simulink model "Wanchao_Shuttlecock_New"  (Simulink 7.7)
settings: Solver=ode4  StartTime=0.0  StopTime=inf  FixedStep=sample_time  RelTol=1e-3
InitFcn:
  | sample_time=0.005;%0.004;%0.0025;%0.02;
  | DeltaT = 0.02;
  | g = 9.81;
  | H0 = g%0.3165;
  | Kl = 1;
  | 
  | Omega_r = 1.6;%for Horizontal reference
  | Zeta_r = 0.7; %for Horizontal reference
  | Omega = 1.8;%for Horizontal Control
  | Zeta = 0.5;    %for Horizontal Control
  | 
  | Omega_h_r = 2.5; %for vertical reference
  | Zeta_h_r = 0.8;  %for vertical reference
  | Omega_h = 2.7;    %for vertical control
  | Zeta_h = 0.8;         %for vertical control
  | PI=pi;
  | 
  | Mass = 1;
  | Acc_Max = 4;
  | Acc_Max_h = 4;
  | 
  | Max_RP = 60;
undefined symbols (not defined in the file or in its folder): DiscIntNeverNeededParam
libraries: simulink x7, dspadpt3 x3, X330_Control x2, X400_Control x1
(part 2 of 2)

== stateflow chart Planning/Trajectory Logic/UAV SF ==
  state Airborne
    state TakeOff
      du:HoverThrottle = (H0 - HoverThrottle)*3*DeltaT + HoverThrottle ;
    state Initialization
      du:PosDesired[0]=InitialPos[0];PosDesired[1]=InitialPos[1];
      PosDesired[2]=InitialPos[2];
    state SafyHover
      en:PosDesired = Pos; PosDesired[2]=-0.9;
    state Prelanding
      en:PosDesired[0]=InitialPos[0];PosDesired[1]=InitialPos[1];
      PosDesired[2]=InitialPos[2];
    state Descent
      en:PosDesired[2] = PerchPos[2]-0.15;
    state TrajE
      state OutputTargetPos
        en:PosDesired[0]=xp;
        PosDesired[1]=yp;
        PosDesired[2]=zp;
        dp[0]=xp;dp[1]=yp;dp[2]=zp;
      state DAQ
        en:i=0;DataReady=0;
        du:x[i]=Shuttlecock[0];[i]=Shuttlecock[1];
        z[i]=Shuttlecock[2];i++;
      state Estimation
        en:[xp,yp,zp,drz,rr]=TrajEst2(x,y,z,H);
      OutputTargetPos -> (junction 26)
      (default) -> DAQ
      Estimation -> OutputTargetPos [order 2] : [(abs(xp)<1)&(abs(yp+0.5)<1)]
      Estimation -> (junction 26) [order 1] : [(abs(xp)>=1)|(abs(yp+0.5)>=1)]
      DAQ -> Estimation : [i==5]
      (junction 26) -> DAQ [order 2] : [(Shuttlecock[2]-H<=-0.4)|(drz<0)]
    (default) -> TakeOff : {PosDesired = Pos;PosDesired[2] =-0.9;}
    TakeOff -> Initialization : after(1,sec)
    Initialization -> TrajE [order 1] : [(abs(Shuttlecock[0])<1)&(Shuttlecock[1]<2.5)&(Shuttlecock[2]<H-0.2)]
    Initialization -> SafyHover [order 2] : [RC[5] > 0]
    (junction 26) -> SafyHover [order 1] : [(RC[5] > 0)|((Shuttlecock[2]-H>-0.4)&(drz>=0))]
    SafyHover -> Prelanding : after(3, sec)
    Prelanding -> Descent : [PerchError < 0.01]
  state Landing
    state Descending
      en:PosDesired = Pos;
      du:PosDesired[2] = (PerchPos[2]- PosDesired[2])*1*DeltaT + PosDesired[2] ;
    state CutThrottle
      du:HoverThrottle = (0 - HoverThrottle)*3*DeltaT + HoverThrottle ;
    (default) -> Descending
    Descending -> CutThrottle : [Pos[2] > (PerchPos[2]-0.1)]
  (default) -> Airborne : {HoverThrottle = 0;}
  Landing -> Airborne : [RC[6] > 0.5]
  Airborne -> Landing : [RC[6] < -0.5]
  data: px function_input double size=5; py function_input double size=5; pz function_input double size=5; xe function_output double size=1; Hz function_input double size=1; ye function_output double size=1; ze function_output double size=1; zd function_output double size=1; p local double size=3 =[0 0 0]; t constant double size=5 =[0 0.02 0.04 0.06 0.08]; r function_output double; px function_input double size=5; py function_input double size=5; pz function_input double size=5; xe function_output double size=1; Hz function_input double size=1; ye function_output double size=1; ze function_output double size=1; zd function_output double size=1; x local double size=5 =[0 0 0 0 0]; y local double size=5 =[0 0 0 0 0]; z local double size=5 =[0 0 0 0 0]; xp local double; yp local double; zp local double; x_cache local double size=5 =[0 0 0 0 0]; y_cache local double size=5 =[0 0 0 0 0]; z_cache local double size=5 =[0 0 0 0 0]; px function_input double size=5; py function_input double size=5; pz function_input double size=5; xe function_output double size=1; Hz function_input double size=1; ye function_output double size=1; ze function_output double size=1; zd function_output double size=1; PosDesired output double size=4; HoverThrottle output double size=1; Mode output uint8 size=1; RC input double size=8; Pos input double size=4; PerchPos input double size=4; DeltaT parameter double size=1; H0 parameter double size=1; Kl parameter double size=1; VelCmd local double size=2 =0; PWM output double; PerchError input double; PI parameter double size=1; Shuttlecock input double size=3; H constant double =-1; InitialPos constant double size=3 =[0 -0.5 -0.9]; i local double =0; dp output double size=3 =[0 0 0]; drz local double; a local double; b local double; c local double; rr local double
  function [xe,ye,ze,zd,r]=TrajEst2(px,py,pz,Hz):
    | function [xe,ye,ze,zd,r]=TrajEst2(px,py,pz,Hz)
    | 
    | zd=sign(pz(end)-pz(1));
    | 
    | p=polyfit(t,pz,2)';
    | a=p(1);
    | b=p(2);
    | c=p(3);
    | r=b^2-4*a*(c-Hz);
    | if r>=0
    |     te=(-b+sqrt(r))/(2*a);
    |     xe=polyval(polyfit(t,px,1),te);
    |     ye=polyval(polyfit(t,py,1),te);
    | else
    |     xe=0;
    |     ye=-2;
    | end
    | ze=Hz;
  function [xe,ye,ze,zd]=TrajEst(px,py,pz,Hz):
    | function [xe,ye,ze,zd]=TrajEst(px,py,pz,Hz)
    | 
    | sgn=sign(mean(diff(px)));
    | zd=sign(pz(5)-pz(4));
    | dx=sgn*0.01;
    | x=-1:0.02:1;
    | y=0.5:-0.01:-1.5;
    | 
    | tr_zx=polyval(polyfit(px,pz,2),x);
    | tr_zy=polyval(polyfit(py,pz,2),y);
    | 
    | [~,kx]=min(abs(tr_zx-Hz));
    | [~,ky]=min(abs(tr_zy-Hz));
    | 
    | xe=x(kx);
    | ye=y(ky);
    | ze=Hz;
  function [xe,ye,ze,zd]=TrajEst1(px,py,pz,Hz):
    | function [xe,ye,ze,zd]=TrajEst1(px,py,pz,Hz)
    | 
    | zd=sign(pz(5)-pz(4));
    | 
    | p=polyfit(py,pz,2);
    | a=p(1);
    | b=p(2);
    | c=p(3);
    | r=b^2-4*a*(c-Hz);
    | if r>=0
    |    ye=(-b+sqrt(r))/(2*a);
    | else
    |     ye=0;
    | end
    | 
    | p=polyfit(px,pz,2);
    | a=p(1);
    | b=p(2);
    | c=p(3);
    | r=b^2-4*a*(c-Hz);
    | if r>=0
    |    xe=(-b+sqrt(r))/(2*a);
    | else
    |    xe=0;
    | end
    | 
    | ze=Hz;
